simulink model "vkr_ch2_sync"  (R2025b)
settings: Solver=FixedStepDiscrete  StartTime=0.0  StopTime=Nsym/Rs  FixedStep=1/Fs_tx  RelTol=1e-3
values from neighbouring files (symbols this model uses):
  Fs_tx = Rs * sps_tx    (= 8000000)    [params_tx.m]    (also in test_sync_loop.m)
  k_bits = log2(M)    [compare_all_architectures.m]    (also in compare_round_period_ber.m; compare_sync_direct.m; params_tx.m; run_ber_curve.m)
  Nsym = 10000    [params_tx.m]    (also in run_dynamics.m = 3000; run_sco_test.m = 30000; test_modelsim_io.m = 5000; test_rice_loop.m = 5000)
  rolloff = 0.35    [compare_all_architectures.m]    (also in compare_round_period_ber.m; compare_sync_direct.m; params_tx.m; process_real_data.m = 0.2)
  Rs = 1e6    (= 1000000)    [params_tx.m]    (also in test_sync_loop.m)
  sps_tx = 40    [compare_all_architectures.m]    (also in compare_round_period_ber.m; compare_sync_direct.m = 8; params_tx.m = 8; run_ber_curve.m = 8)
  timing_offset = 0.3    [compare_all_architectures.m]    (also in compare_round_period_ber.m; compare_sync_direct.m; params_tx.m; run_ber_curve.m)
libraries: commfilt2 x2, commchan3 x1, commrandsrc3 x1, commdigbbndpm3 x1, commsync2 x1, dspsigops x1
settings Model: Creator=Gostie2k  LastModifiedBy=t-kudimov

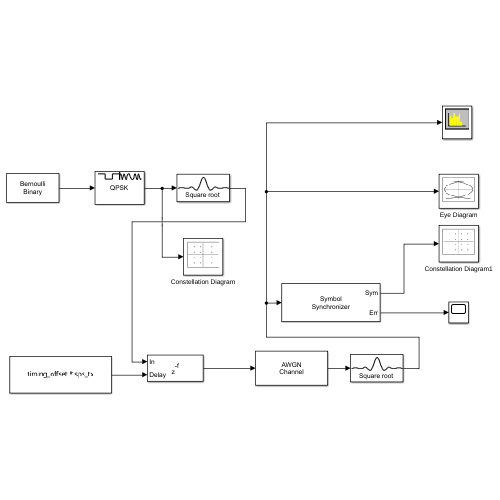
[thumbnail: Simulink's stored preview of the top-level diagram]
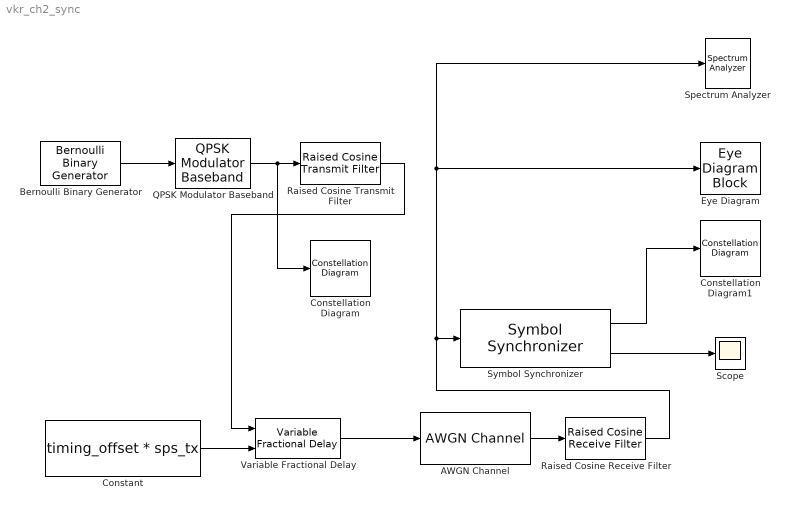
== system vkr_ch2_sync ==
  AWGN Channel : commchan3/AWGN Channel  LegacyMode=off  NoiseMethod="Signal to noise ratio  (Eb/No)"  noiseMode="Signal to noise ratio  (SNR)"  EbNo=EbNo_dB  EsNo=10  SNR=10  BitsPerSymbol=k_bits  SignalPower=1  SpecifySymbolPeriod=off  SamplesPerSymbol=sps_tx  SymbolPeriod=1  VarianceSource=Parameter  Variance=1  RandomStream=Global stream  Seed=67  SimulateUsing=Code generation
  Bernoulli Binary Generator : commrandsrc3/Bernoulli Binary Generator  ProbabilityOfZero=0.5  SeedSource=Parameter  Seed=12345  SampleTime=1/(Rs*k_bits)  SamplesPerFrame=k_bits*Nsym  OutputDataType=double  SimulateUsing=Interpreted execution
  Constant : Constant  Value=timing_offset * sps_tx  OutDataTypeStr=double  SampleTime=1/Fs_tx
  Constellation Diagram : ConstellationDiagram  WindowPosition=[481.000000,385.000000,600.000000,605.000000,]  ScopeFrameLocation=window  ShowLegend=on
  Constellation Diagram1 : ConstellationDiagram  WindowPosition=[74.000000,-277.000000,600.000000,605.000000,]  ScopeFrameLocation=window  ShowLegend=on
  Eye Diagram : EyeDiagramBlock  WindowPosition=[1527.000000,-530.000000,1440.000000,749.000000,]  ScopeFrameLocation=window  SamplesPerSymbol=2  TracesToDisplay=200  ColorFading=on
  QPSK Modulator Baseband : commdigbbndpm3/QPSK Modulator Baseband  InType=Bit  Enc=Gray  Ph=pi/4  outDtype=double  outWordLen=16  outUDDataType=sfix(16)  outFracLenMode=Best precision  outFracLen=15  outDataTypeStr=double  outLastDataTypeStr=double
  Raised Cosine Receive Filter : commfilt2/Raised Cosine Receive Filter  filtType=Square root  R=rolloff  filtSpan=span  N=sps_tx  downFactor=decim  downOffset=0  filterGain=1/sqrt(sps_tx)  InputProcessing=Columns as channels (frame based)  RateOptions=Allow multirate processing  framing=Mute  checkCoeff=off  variableName=rcRxFilt  currentFiltSpan=10  D=5  inputOffset=0  sampMode=Mute  saveAsFlag=0  rateMode=Downsampling  checkGain=Normalized  launchFVT=on  roundingMode=Floor  overflowMode=off  coeffDataTypeStr=Inherit: Same word length as input  coeffMin=[]  coeffMax=[]  coeffLastDataTypeStr=Inherit: Same word length as input  accumDataTypeStr=Inherit: Same as product output  accumLastDataTypeStr=Inherit: Same as product output  outputDataTypeStr=Inherit: Same as accumulator  outputMin=[]  outputMax=[]  outputLastDataTypeStr=Inherit: Same as accumulator
  Raised Cosine Transmit Filter : commfilt2/Raised Cosine Transmit Filter  filtType=Square root  R=rolloff  filtSpan=span  N=sps_tx  filterGain=sqrt(sps_tx)  InputProcessing=Columns as channels (frame based)  RateOptions=Enforce single-rate processing  framing=Mute  checkCoeff=off  variableName=rcTxFilt  checkGain=Normalized  sampMode=Mute  saveAsFlag=0  currentFiltSpan=10  D=(10)/2  launchFVT=on  roundingMode=Floor  overflowMode=off  coeffDataTypeStr=Inherit: Same word length as input  coeffMin=[]  coeffMax=[]  coeffLastDataTypeStr=Inherit: Same word length as input  outputDataTypeStr=Inherit: Same as accumulator  outputMin=[]  outputMax=[]  outputLastDataTypeStr=Inherit: Same as accumulator
  Scope : Scope
  Spectrum Analyzer : SpectrumAnalyzer  WindowPosition=[1081.000000,-530.000000,1920.000000,1011.000000,]  ScopeFrameLocation=window  SampleRateSource=Property  SampleRate=Fs_tx  WindowInvariantSamplesPerUpdate=on  Span=8000000  StartFrequency=-4000000  StopFrequency=4000000  MaximizeAxes=On  YLimits=[-93.99988261601567 17.831117383984306]
  Symbol Synchronizer : commsync2/Symbol Synchronizer  Modulation=PAM/PSK/QAM  TimingErrorDetector=Gardner (non-data-aided)  SamplesPerSymbol=sps_rx  DampingFactor=zeta  NormalizedLoopBandwidth=BnT  DetectorGain=2.7  TimingErrorOutputPort=on  SimulateUsing=Code generation
  Variable Fractional Delay : dspsigops/Variable Fractional Delay  mode=OBSOLETE  modeActive=FIR  L=4  FarrowL=4  R=10  alpha=1  dmax=32  InputProcessing=Columns as channels (frame based)  ic=0  noDFT=off  fallbackFIR=Clip to the minimum value necessary for centered kernel  fallbackFarrow=Clip to the minimum value necessary for centered kernel  roundingMode=Zero  overflowMode=off
  wires:
  Variable Fractional Delay/1 -> AWGN Channel/1
  Bernoulli Binary Generator/1 -> QPSK Modulator Baseband/1
  QPSK Modulator Baseband/1 -> Constellation Diagram/1, Raised Cosine Transmit Filter/1
  Constant/1 -> Variable Fractional Delay/2
  AWGN Channel/1 -> Raised Cosine Receive Filter/1
  Raised Cosine Transmit Filter/1 -> Variable Fractional Delay/1
  Raised Cosine Receive Filter/1 -> Spectrum Analyzer/1, Eye Diagram/1, Symbol Synchronizer/1
  Symbol Synchronizer/2 -> Scope/1
  Symbol Synchronizer/1 -> Constellation Diagram1/1
